simulink model "model"  (R2021a)
settings: Solver=ode4  StartTime=0.0  StopTime=4  FixedStep=tA  RelTol=1e-3
values from neighbouring files (symbols this model uses):
  c = [65536*vmax*vmax*vmax*vmax*vmax /(xs*xs*xs*xs*253125);      -4096*vmax*vmax*vmax*vmax / (xs*xs*xs*3375);      1024*vmax*vmax*vmax / (xs*xs*675);      0;      0;      x0]    [cd_refpoly_vmax.m]
  cff = [c(1);        c(2) + 5*c(1)*a1;        c(3) + 4*c(2)*a1 + 20*c(1)*a2;        c(4) + 3*c(3)*a1 + 12*c(2)*a2 + 60*c(1)*a3;        c(5) + 2*c(4)*a1 +  6*c(3)*a2 + 24*c(2)*a3;        c(6) +   c(5)*a1 +  2*c(4)*a2 +  6*c(3)*a3]    [cd_refpoly_ff.m]    (also in ex6_1.m = cd_refpoly_ff(c, k, T, Tt, kr, Ti))
  te = 15 * xs / (8 * vmax)    [cd_refpoly_vmax.m]
  xs = 1    [ex6_1.m]
libraries: cstblocks x4
settings Model: Creator=matti  LastModifiedBy=matti

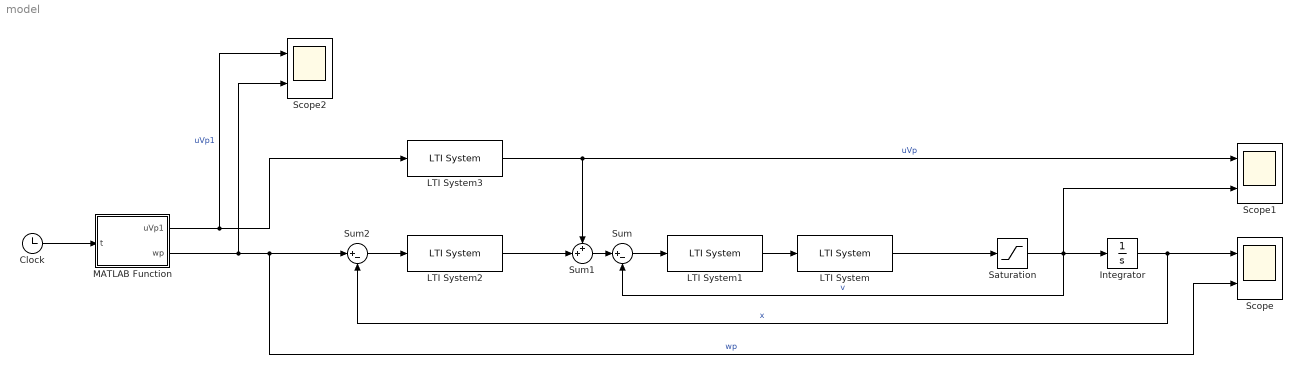
== system model ==
  Clock : Clock
  Integrator : Integrator
  LTI System : cstblocks/LTI System  sys=G_S  IC=[]
  LTI System1 : cstblocks/LTI System  sys=G_R  IC=[]
  LTI System2 : cstblocks/LTI System  sys=G_Rp  IC=[]
  LTI System3 : cstblocks/LTI System  sys=G_Vp1  IC=[]
  MATLAB Function : MATLAB Function  TreatAsAtomicUnit=on
  Saturation : Saturate  UpperLimit=1  LowerLimit=-1
  Scope : Scope  NumInputPorts=2
  Scope1 : Scope  NumInputPorts=2
  Scope2 : Scope  NumInputPorts=2
  Sum : Sum  Inputs=|+-
  Sum1 : Sum  Inputs=++|
  Sum2 : Sum  Inputs=|+-
  wires:
  LTI System1/1 -> LTI System/1
  Integrator/1 -> Scope/1, Sum2/2  "x"
  Sum1/1 -> Sum/1
  Sum/1 -> LTI System1/1
  LTI System2/1 -> Sum1/2
  LTI System3/1 -> Sum1/1, Scope1/1  "uVp"
  Sum2/1 -> LTI System2/1
  MATLAB Function/2(wp) -> Scope2/2, Scope/2, Sum2/1  "wp"
  MATLAB Function/1(uVp1) -> Scope2/1, LTI System3/1  "uVp1"
  Saturation/1 -> Scope1/2, Integrator/1, Sum/2  "v"
  Clock/1 -> MATLAB Function/1(t)
  LTI System/1 -> Saturation/1

== matlab function model/MATLAB Function ==
  data: uVp1 output; wp output; t input; c parameter; cff parameter; te parameter; xs parameter
function [uVp1, wp] = fcn(t, c, cff, te, xs)
if t < te
    uVp1 = cff(1) * t^5 + cff(2) * t^4 + cff(3) * t^3 + cff(4) * t^2 + cff(5) * t + cff(6);
    wp = c(1) * t^5 + c(2) * t^4 + c(3) * t^3 + c(4) * t^2 + c(5) * t + c(6);
else
    uVp1 = xs;
    wp = xs;
end
